simulink model "Es56"  (R2021b)
settings: Solver=VariableStepAuto  StartTime=0.0  StopTime=3  FixedStep=1e-3  RelTol=1e-5
undefined symbols (not defined in the file or in its folder): Kd_ws, Kp_ws, Orientation, p560_nofric, Position_End_effector, rho, Velocity
libraries: roblocks x6
settings Model: Creator=Andrea  LastModifiedBy=mular
settings SolverCC: AlgebraicLoopSolver=TrustRegion
settings DataIOCC: ReturnWorkspaceOutputs=off
settings DebuggingCC: SFMachineParentedDataDiag=warning  ArithmeticOperatorsInVariantConditions=warning
settings SFSimCC: CustomCodeUndefinedFunction=UseInterfaceOnly

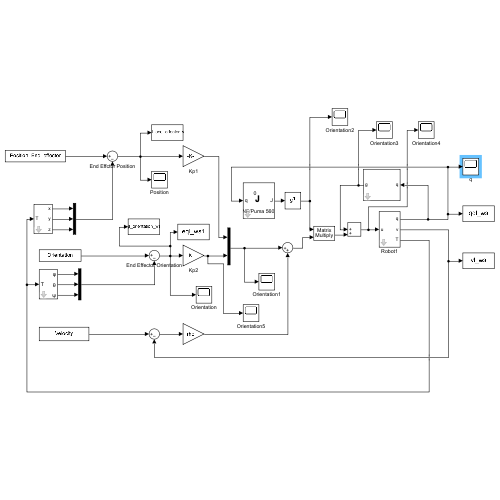
[thumbnail: Simulink's stored preview of the top-level diagram]
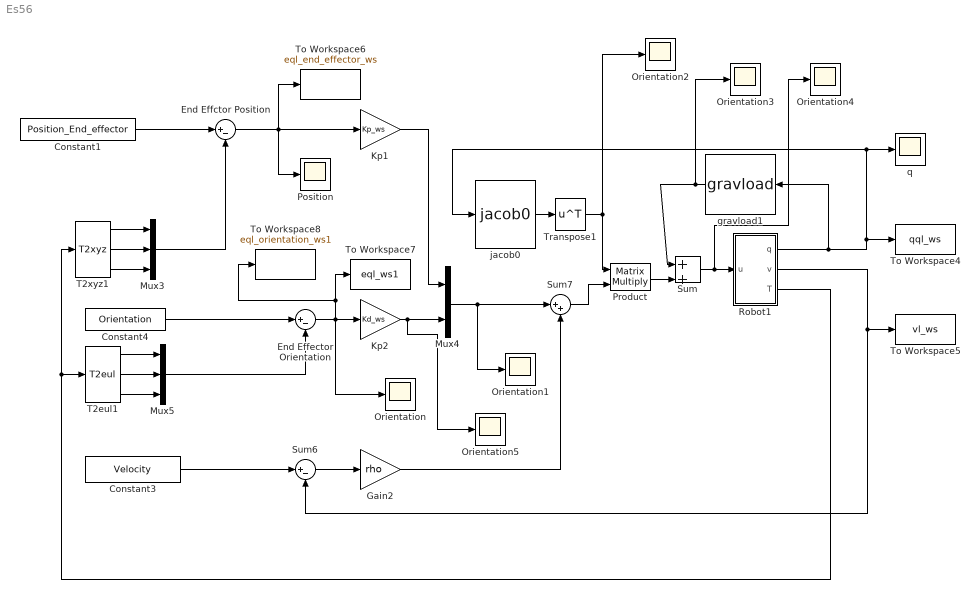
== system Es56 ==
  Constant1 : Constant  Value=Position_End_effector
  Constant3 : Constant  Value=Velocity
  Constant4 : Constant  Value=Orientation
  End Effctor Position : Sum  Inputs=|+-
  End Effector Orientation : Sum  Inputs=|+-
  Gain2 : Gain  Gain=rho
  Kp1 : Gain  Gain=Kp_ws
  Kp2 : Gain  Gain=Kd_ws
  Mux3 : Mux  Inputs=3
  Mux4 : Mux  Inputs=2
  Mux5 : Mux  Inputs=3
  Orientation{,1..5} (6 alike) : Scope
  Position : Scope
  Product : Product  Multiplication=Matrix(*)
  Robot1 : Subsystem  mask{robot=p560_nofric, q0=[0 0 0 0 pi/2 0]}
      mask prompts: robot "Robot object"; q0 "Initial state"
  Sum : Sum  Inputs=|++
  Sum6 : Sum  Inputs=|+-
  Sum7 : Sum  Inputs=|++
  T2eul1 : roblocks/Toolbox/T2eul  degrees=off
  T2xyz1 : roblocks/Toolbox/T2xyz
  To Workspace4 : ToWorkspace  VariableName=qql_ws  SaveFormat=Timeseries  SampleTime=-1
  To Workspace5 : ToWorkspace  VariableName=vl_ws  SampleTime=-1
  To Workspace6 : ToWorkspace  VariableName=eql_end_effector_ws  SampleTime=-1
  To Workspace7 : ToWorkspace  VariableName=eql_ws1  SampleTime=-1
  To Workspace8 : ToWorkspace  VariableName=eql_orientation_ws1  SampleTime=-1
  Transpose1 : Math  Operator=transpose  SaturateOnIntegerOverflow=on
  gravload1 : roblocks/Arm/gravload  robot=p560_nofric
  "jacob0 " : roblocks/Arm/jacob0   robot=p560_nofric
      link override MATLAB Fcn: MATLABFcn=jacob0(robot,u, 'eul')
  q : Scope
  wires:
  gravload1/1 -> Sum/1, Orientation3/1
  Robot1/2(v) -> To Workspace5/1, Sum6/2
  Constant4/1 -> End Effector Orientation/1
  T2xyz1/3 -> Mux3/3
  Gain2/1 -> Sum7/2
  Sum7/1 -> Product/2
  T2xyz1/1 -> Mux3/1
  Constant1/1 -> End Effctor Position/1
  Constant3/1 -> Sum6/1
  Sum6/1 -> Gain2/1
  T2eul1/2 -> Mux5/2
  Transpose1/1 -> Product/1, Orientation2/1
  Mux4/1 -> Orientation1/1, Sum7/1
  T2eul1/3 -> Mux5/3
  Robot1/3(T) -> T2xyz1/1, T2eul1/1
  "jacob0 "/1 -> Transpose1/1
  End Effctor Position/1 -> Position/1, Kp1/1, To Workspace6/1
  Kp1/1 -> Mux4/1
  Mux3/1 -> End Effctor Position/2
  T2eul1/1 -> Mux5/1
  Kp2/1 -> Orientation5/1, Mux4/2
  End Effector Orientation/1 -> To Workspace7/1, To Workspace8/1, Orientation/1, Kp2/1
  T2xyz1/2 -> Mux3/2
  Mux5/1 -> End Effector Orientation/2
  Robot1/1(q) -> "jacob0 "/1, q/1, To Workspace4/1, gravload1/1
  Sum/1 -> Orientation4/1, Robot1/1(u)
  Product/1 -> Sum/2

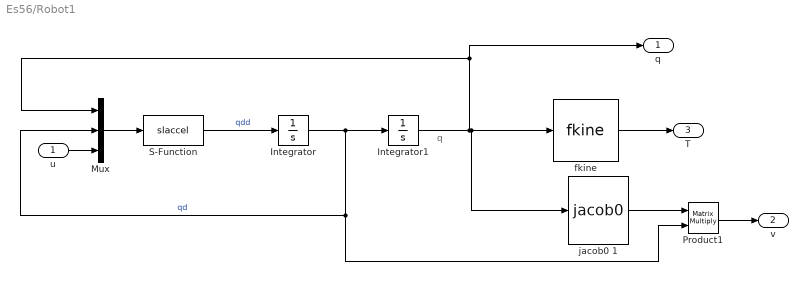
== system Es56/Robot1 ==
  note: q
  u : Inport
  Integrator : Integrator
  Integrator1 : Integrator  InitialCondition=q0
  Mux : Mux  Inputs=3
  Product1 : Product  Multiplication=Matrix(*)
  S-Function : S-Function  FunctionName=slaccel  Parameters=p560_nofric  SFunctionDeploymentMode=off  EnableBusSupport=off
  fkine : roblocks/Arm/fkine  robot=p560_nofric
  jacob0 1 : roblocks/Arm/jacob0   robot=p560_nofric
      link override MATLAB Fcn: MATLABFcn=jacob0(robot,u, 'eul')
  q : Outport  VectorParamsAs1DForOutWhenUnconnected=off
  v : Outport  Port=2  VectorParamsAs1DForOutWhenUnconnected=off
  T : Outport  Port=3  VectorParamsAs1DForOutWhenUnconnected=off
  wires:
  S-Function/1 -> Integrator/1  "qdd"
  Mux/1 -> S-Function/1
  Integrator/1 -> Product1/2, Mux/2, Integrator1/1  "qd"
  u/1 -> Mux/3
  Integrator1/1 -> q/1, Mux/1, fkine/1, jacob0 1/1
  jacob0 1/1 -> Product1/1
  Product1/1 -> v/1
  fkine/1 -> T/1
